simulink model "LAB2_motorDC_VI"  (Simulink 9.2)
settings: Solver=ode5  StartTime=0.0  StopTime=4  FixedStep=1e-3  RelTol=1e-6  EnableMultiTasking=on
InitFcn:
  | main_STR_no_canc;
values from neighbouring files (symbols this model uses):
  b = 2.4299e-004    (= 0.00024299)    [main_STR_no_canc.m]
  denHu = [1 0]    [main_STR_no_canc.m]
  denHy = denHu    [main_STR_no_canc.m]
  J = Jm+Jd1    (= 3.78e-05)    [main_STR_no_canc.m]
  Kd = a * sin( alpha )/w_co    [4.2.m]    (also in part4_2.m)
  Kd_b = a_b * sin( alpha_b )/w_co    [4.2.m]    (also in part4_2.m)
  Ki = 2    [main_STR_no_canc.m]
  Kp = a * cos( alpha )    [4.2.m]    (also in part4_2.m)
  Kp_b = a_b * cos( alpha_b )    [4.2.m]    (also in part4_2.m)
  Kt = 0.071    [main_STR_no_canc.m]
  numHu = 1    [main_STR_no_canc.m]
  numHy = [1 -1]    [main_STR_no_canc.m]
  tau_c = 1/( w_co * 100 )    (= 0.00075)    [4.2.m]    (also in part4_2.m = 0.0075)
  tau_c_b = 1/( w_co * 100)    (= 0.00075)    [4.2.m]    (also in part4_2.m = 0.0075)
  Ts = 0.001    [main_STR_no_canc.m]
libraries: simulink x2
settings Model: Creator=lab  LastModifiedBy=Luca  ExtModeTrigDuration=100000
settings DataIOCC: LimitDataPoints=off
settings OptimizationCC: ExpressionDepthLimit=2147483647
settings DebuggingCC: SolverPrmCheckMsg=warning
settings HardwareCC: ProdIntDivRoundTo=Zero  ProdEndianess=LittleEndian  ProdHWDeviceType=Generic->32-bit x86 compatible
settings SFSimCC: SimParseCustomCode=off
settings RTWCC: SystemTargetFile=rtwin.tlc  TemplateMakefile=rtwin.tmf  Description=Real-Time Windows Target  RTWCompilerOptimization=on
settings CodeAppCC: MaxIdLength=95
settings TargetCC: TargetLibSuffix=_rtwin.lib  TargetPreCompLibLocation=C:\Programmi\matlab\R2009a\toolbox\rtw\targets\rtwin\lib  GeneratePreprocessorConditionals=Use local settings  PreserveStateflowLocalDataDimensions=off
settings CustomProperty: DataType=string

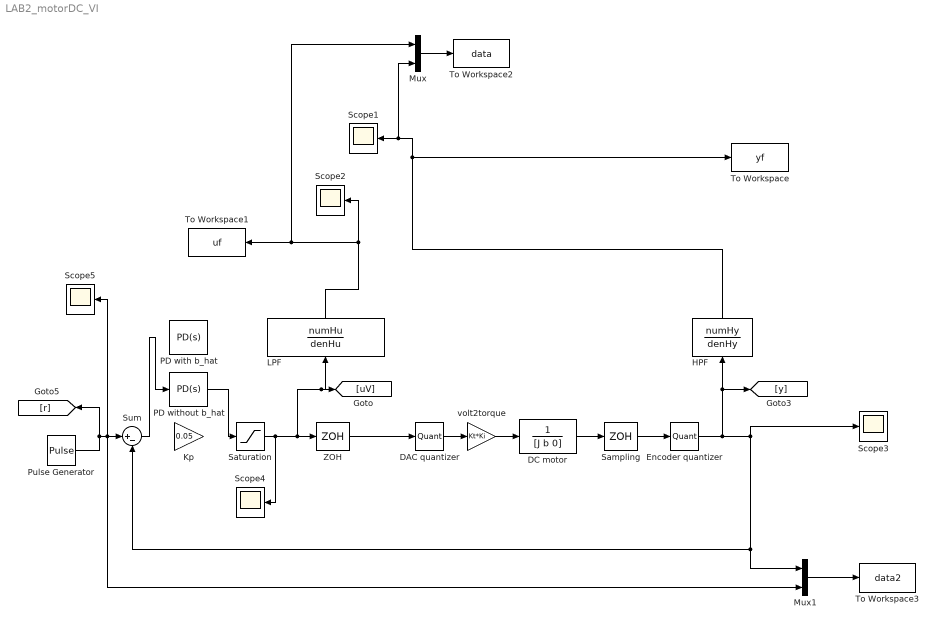
== system LAB2_motorDC_VI ==
  DAC quantizer : Quantizer  QuantizationInterval=10/2^13
  DC motor : TransferFcn  Denominator=[J b 0]
  Encoder quantizer : Quantizer  QuantizationInterval=2*pi/2000
  HPF : DiscreteTransferFcn  Numerator=numHy  Denominator=denHy  SampleTime=Ts
  Kp : Gain  Gain=0.05
  LPF : DiscreteTransferFcn  Numerator=numHu  Denominator=denHu  SampleTime=Ts
  Mux : Mux  Inputs=2
  Mux1 : Mux  Inputs=2
  PD with b_hat : simulink/Continuous/PID Controller  Controller=PD  Form=Parallel  TimeDomain=Continuous-time  SampleTime=-1  IntegratorMethod=Forward Euler  FilterMethod=Forward Euler  ControllerParametersSource=internal  P=Kp_b  I=1  D=Kd_b  UseFilter=on  N=1/tau_c_b  TunerSelectOption=Transfer Function Based (PID Tuner App)  InitialConditionSource=internal  InitialConditionForIntegrator=0  InitialConditionForFilter=0  DifferentiatorICPrevScaledInput=0  ExternalReset=none  TrackingMode=off  Kt=1  LimitOutput=off  UpperSaturationLimit=inf  LowerSaturationLimit=-inf  LinearizeAsGain=on  AntiWindupMode=none  Kb=1  POutMin=[]  POutMax=[]  IOutMin=[]  IOutMax=[]  DOutMin=[]  DOutMax=[]  NOutMin=[]  NOutMax=[]  SumOutMin=[]  SumOutMax=[]  SaturationOutMin=[]  SaturationOutMax=[]  PParamMin=[]  PParamMax=[]  IParamMin=[]  IParamMax=[]  DParamMin=[]  DParamMax=[]  NParamMin=[]  NParamMax=[]  KbParamMin=[]  KbParamMax=[]  KtParamMin=[]  KtParamMax=[]  KbOutMin=[]  KbOutMax=[]  KtOutMin=[]  KtOutMax=[]  IntegratorOutMin=[]  IntegratorOutMax=[]  FilterOutMin=[]  FilterOutMax=[]  SumI1OutMin=[]  SumI1OutMax=[]  SumI2OutMin=[]  SumI2OutMax=[]  SumI3OutMin=[]  SumI3OutMax=[]  SumI4OutMin=[]  SumI4OutMax=[]  SumDOutMin=[]  SumDOutMax=[]  DifferentiatorOutMin=[]  DifferentiatorOutMax=[]  FilterDiffOutCoefMin=[]  FilterDiffOutCoefMax=[]  ReciprocalOutMin=[]  ReciprocalOutMax=[]  SumDenOutMin=[]  SumDenOutMax=[]  SumNumOutMin=[]  SumNumOutMax=[]  DivideOutMin=[]  DivideOutMax=[]  IntegratorContinuousStateAttributes=''  IntegratorStateMustResolveToSignalObject=off  IntegratorRTWStateStorageClass=Auto  FilterContinuousStateAttributes=''  FilterStateMustResolveToSignalObject=off  FilterRTWStateStorageClass=Auto  ParallelPVariant=InternalParameters  IdealPVariant=Disabled  IVariant=Disabled  DVariant=InternalParameters  IntegratorVariant=Disabled  SatVariant=Disabled  AWVariant=Disabled  PCopyVariant=Disabled  TRVariant=Disabled  FdbkBlocksVariant=Forward  IdealPFdbkVariant=Disabled  SatFdbkVariant=Disabled  DerivativeFilterVariant=ContFilter  NVariant=InternalParameters  NCopyVariant=Disabled  FilterICVariant=InternalICsFilter  IntegratorICVariant=Disabled  ExternalResetVariant=Disabled  TRSumVariant=Passthrough  SumFdbkVariant=Disabled  SumVariant=Sum_PD
  PD without b_hat : simulink/Continuous/PID Controller  Controller=PD  Form=Parallel  TimeDomain=Continuous-time  SampleTime=-1  IntegratorMethod=Forward Euler  FilterMethod=Forward Euler  ControllerParametersSource=internal  P=Kp  I=1  D=Kd  UseFilter=on  N=1/tau_c  TunerSelectOption=Transfer Function Based (PID Tuner App)  InitialConditionSource=internal  InitialConditionForIntegrator=0  InitialConditionForFilter=0  DifferentiatorICPrevScaledInput=0  ExternalReset=none  TrackingMode=off  Kt=1  LimitOutput=off  UpperSaturationLimit=inf  LowerSaturationLimit=-inf  LinearizeAsGain=on  AntiWindupMode=none  Kb=1  POutMin=[]  POutMax=[]  IOutMin=[]  IOutMax=[]  DOutMin=[]  DOutMax=[]  NOutMin=[]  NOutMax=[]  SumOutMin=[]  SumOutMax=[]  SaturationOutMin=[]  SaturationOutMax=[]  PParamMin=[]  PParamMax=[]  IParamMin=[]  IParamMax=[]  DParamMin=[]  DParamMax=[]  NParamMin=[]  NParamMax=[]  KbParamMin=[]  KbParamMax=[]  KtParamMin=[]  KtParamMax=[]  KbOutMin=[]  KbOutMax=[]  KtOutMin=[]  KtOutMax=[]  IntegratorOutMin=[]  IntegratorOutMax=[]  FilterOutMin=[]  FilterOutMax=[]  SumI1OutMin=[]  SumI1OutMax=[]  SumI2OutMin=[]  SumI2OutMax=[]  SumI3OutMin=[]  SumI3OutMax=[]  SumI4OutMin=[]  SumI4OutMax=[]  SumDOutMin=[]  SumDOutMax=[]  DifferentiatorOutMin=[]  DifferentiatorOutMax=[]  FilterDiffOutCoefMin=[]  FilterDiffOutCoefMax=[]  ReciprocalOutMin=[]  ReciprocalOutMax=[]  SumDenOutMin=[]  SumDenOutMax=[]  SumNumOutMin=[]  SumNumOutMax=[]  DivideOutMin=[]  DivideOutMax=[]  IntegratorContinuousStateAttributes=''  IntegratorStateMustResolveToSignalObject=off  IntegratorRTWStateStorageClass=Auto  FilterContinuousStateAttributes=''  FilterStateMustResolveToSignalObject=off  FilterRTWStateStorageClass=Auto  ParallelPVariant=InternalParameters  IdealPVariant=Disabled  IVariant=Disabled  DVariant=InternalParameters  IntegratorVariant=Disabled  SatVariant=Disabled  AWVariant=Disabled  PCopyVariant=Disabled  TRVariant=Disabled  FdbkBlocksVariant=Forward  IdealPFdbkVariant=Disabled  SatFdbkVariant=Disabled  DerivativeFilterVariant=ContFilter  NVariant=InternalParameters  NCopyVariant=Disabled  FilterICVariant=InternalICsFilter  IntegratorICVariant=Disabled  ExternalResetVariant=Disabled  TRSumVariant=Passthrough  SumFdbkVariant=Disabled  SumVariant=Sum_PD
  Pulse Generator : DiscretePulseGenerator  PulseType=Time based  Amplitude=(360 * 5 + 90) * pi/180  Period=8  PulseWidth=50  PhaseDelay=1
  Sampling : ZeroOrderHold  SampleTime=Ts
  Saturation : Saturate  UpperLimit=3  LowerLimit=-3
  Scope{1..5} (5 alike) : Scope
  Sum : Sum  Inputs=|+-
  To Workspace : ToWorkspace  VariableName=yf  SaveFormat=Timeseries  SampleTime=-1
  To Workspace1 : ToWorkspace  VariableName=uf  SaveFormat=Timeseries  SampleTime=-1
  To Workspace2 : ToWorkspace  VariableName=data  SaveFormat=Structure With Time  SampleTime=-1
  To Workspace3 : ToWorkspace  VariableName=data2  SaveFormat=Structure With Time  SampleTime=-1
  ZOH : ZeroOrderHold  SampleTime=Ts
  volt2torque : Gain  Gain=Kt*Ki
  wires:
  Pulse Generator/1 -> Mux1/2, Scope5/1, Sum/1, [r]
  Sum/1 -> PD without b_hat/1
  DC motor/1 -> Sampling/1
  volt2torque/1 -> DC motor/1
  Sampling/1 -> Encoder quantizer/1
  ZOH/1 -> DAC quantizer/1
  DAC quantizer/1 -> volt2torque/1
  LPF/1 -> Mux/1, To Workspace1/1, Scope2/1
  Encoder quantizer/1 -> Mux1/1, Sum/2, Scope3/1, HPF/1, [y]
  HPF/1 -> To Workspace/1, Mux/2, Scope1/1
  Saturation/1 -> Scope4/1, LPF/1, [uV], ZOH/1
  Mux/1 -> To Workspace2/1
  PD without b_hat/1 -> Saturation/1
  Mux1/1 -> To Workspace3/1
